simulink model "function_caller"  (R2024b)
settings: Solver=VariableStepAuto  StartTime=0.0  StopTime=10.0  RelTol=1e-3
libraries: simulink x1
settings Model: Creator=Ahmad  LastModifiedBy=Ahmad

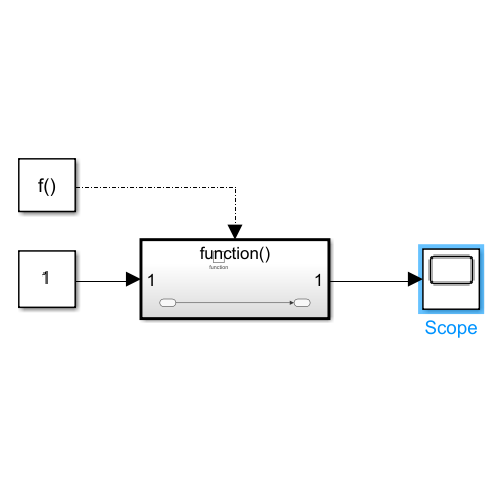
[thumbnail: Simulink's stored preview of the top-level diagram]
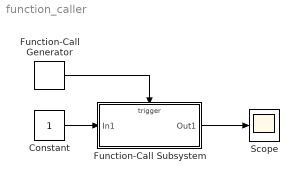
== system function_caller ==
  Constant : Constant
  Function-Call Generator : simulink/Ports & Subsystems/Function-Call Generator  sample_time=0.5  numberOfIterations=1  DisallowWideOutput=off
  Function-Call Subsystem : Subsystem  TreatAsAtomicUnit=on
  Scope : Scope
  wires:
  Function-Call Subsystem/1(Out1) -> Scope/1
  Constant/1 -> Function-Call Subsystem/1(In1)
  Function-Call Generator/1 -> Function-Call Subsystem/Trigger

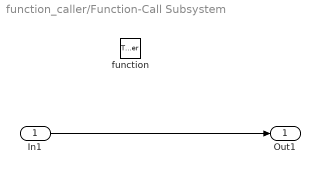
== system function_caller/Function-Call Subsystem ==
  In1 : Inport
  function : TriggerPort  TriggerType=function-call  VariantControl=(inherit)
  Out1 : Outport
  wires:
  In1/1 -> Out1/1
